simulink model "trainGate"  (R2014b)
settings: Solver=FixedStepDiscrete  StartTime=0.0  StopTime=100000  FixedStep=0.01  MaxStep=0.0001  RelTol=1e-3
settings Model: Creator=sand080  LastModifiedBy=sand080
settings DataIOCC: LimitDataPoints=off

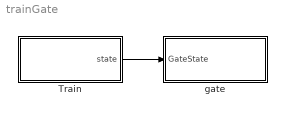
== system trainGate ==
  Train : Subsystem
  gate : Subsystem
  wires:
  Train/1(state) -> gate/1(GateState)

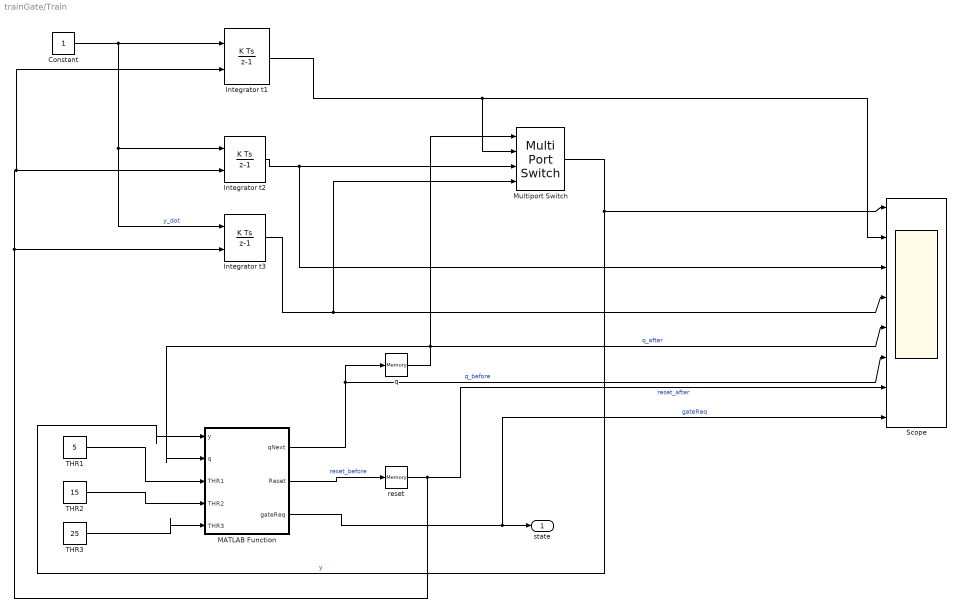
== system trainGate/Train ==
  Constant : Constant
  Integrator t1 : DiscreteIntegrator  ExternalReset=either  InitialConditionSetting=State (most efficient)  SampleTime=-1
  Integrator t2 : DiscreteIntegrator  ExternalReset=either  InitialCondition=5  InitialConditionSetting=State (most efficient)  SampleTime=-1
  Integrator t3 : DiscreteIntegrator  ExternalReset=either  InitialCondition=15  InitialConditionSetting=State (most efficient)  SampleTime=-1
  MATLAB Function : MATLAB Function  Priority=1  TreatAsAtomicUnit=on
  Multiport Switch : MultiPortSwitch
  Scope : Scope  NumInputPorts=8
      settings: TickLabels=on  ShowLegends=on  YMin=0~0~0~10~1~1~0~-1  YMax=40~20~20~30~3~3~1~1
  THR1 : Constant  Value=5
  THR2 : Constant  Value=15
  THR3 : Constant  Value=25
  q : Memory  X0=1  LinearizeMemory=on
  reset : Memory  X0=1  LinearizeMemory=on
  state : Outport
  wires:
  MATLAB Function/1(qNext) -> q/1, Scope/6  "q_before"
  Constant/1 -> Integrator t2/1, Integrator t3/1, Integrator t1/1  "y_dot"
  Integrator t2/1 -> Multiport Switch/3, Scope/3
  Integrator t1/1 -> Scope/2, Multiport Switch/2
  THR1/1 -> MATLAB Function/3(THR1)
  THR2/1 -> MATLAB Function/4(THR2)
  q/1 -> Multiport Switch/1, MATLAB Function/2(q), Scope/5  "q_after"
  THR3/1 -> MATLAB Function/5(THR3)
  Integrator t3/1 -> Multiport Switch/4, Scope/4
  MATLAB Function/2(Reset) -> reset/1  "reset_before"
  Multiport Switch/1 -> Scope/1, MATLAB Function/1(y)  "y"
  reset/1 -> Integrator t1/2, Integrator t2/2, Integrator t3/2, Scope/7  "reset_after"
  MATLAB Function/3(gateReq) -> Scope/8, state/1  "gateReq"

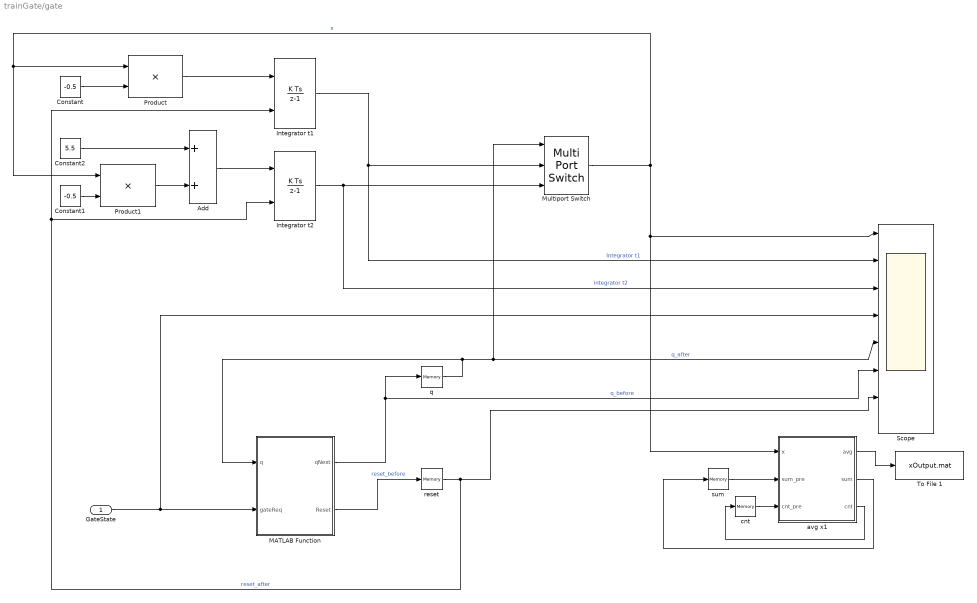
== system trainGate/gate ==
  GateState : Inport
  Add : Sum
  Constant : Constant  Value=-0.5
  Constant1 : Constant  Value=-0.5
  Constant2 : Constant  Value=5.5
  Integrator t1 : DiscreteIntegrator  ExternalReset=either  InitialCondition=10  InitialConditionSetting=State (most efficient)  SampleTime=-1
  Integrator t2 : DiscreteIntegrator  ExternalReset=either  InitialCondition=1  InitialConditionSetting=State (most efficient)  SampleTime=-1
  MATLAB Function : MATLAB Function  Priority=1  TreatAsAtomicUnit=on
  Multiport Switch : MultiPortSwitch  Inputs=2
  Product : Product
  Product1 : Product
  Scope : Scope  NumInputPorts=8
      settings: TickLabels=on  ShowLegends=on  YMin=0~-50~0~-1~1~1~0~-1  YMax=20~50~100~1~2~2~1~1
  To File 1 : ToFile  Filename=xOutput.mat
      settings: Decimation=10000000
  avg x1 : MATLAB Function  Priority=4  TreatAsAtomicUnit=on
  cnt : Memory
  q : Memory  X0=1  LinearizeMemory=on
  reset : Memory  LinearizeMemory=on
  sum : Memory
  wires:
  MATLAB Function/1(qNext) -> q/1, Scope/6  "q_before"
  avg x1/2(sum) -> sum/1
  avg x1/3(cnt) -> cnt/1
  cnt/1 -> avg x1/3(cnt_pre)
  sum/1 -> avg x1/2(sum_pre)
  avg x1/1(avg) -> To File 1/1
  Integrator t2/1 -> Scope/3, Multiport Switch/3  "integrator t2"
  Integrator t1/1 -> Multiport Switch/2, Scope/2  "Integrator t1"
  q/1 -> Multiport Switch/1, Scope/5, MATLAB Function/1(q)  "q_after"
  MATLAB Function/2(Reset) -> reset/1  "reset_before"
  Multiport Switch/1 -> avg x1/1(x), Scope/1, Product/1, Product1/1  "x"
  reset/1 -> Integrator t2/2, Integrator t1/2, Scope/7  "reset_after"
  Constant/1 -> Product/2
  Product/1 -> Integrator t1/1
  Constant1/1 -> Product1/2
  Product1/1 -> Add/2
  Constant2/1 -> Add/1
  Add/1 -> Integrator t2/1
  GateState/1 -> Scope/4, MATLAB Function/2(gateReq)

== matlab function trainGate/gate/MATLAB Function ==
  data: q input; qNext output; Reset output; gateReq input
function [qNext,Reset] = phi(q, gateReq)
%#codegen
if q==1 && gateReq~=1
    qNext=1;
    Reset=0;
elseif q==1 && gateReq==1
    qNext=2;
    Reset=1;
elseif q==2 && gateReq~=-1
    qNext=2;
    Reset=0;
elseif q==2 && gateReq==-1
    qNext=1;
    Reset=1;
else
    qNext=-1; %this should never execute
    Reset=-1; %this should never execute
end

== matlab function trainGate/Train/MATLAB Function ==
  data: y input; q input; qNext output; THR1 input; THR2 input; THR3 input; Reset output; gateReq output
function [qNext,Reset,gateReq] = phi(y,q, THR1, THR2, THR3)
%#codegen
if q==1 && y < THR1
    qNext=1;
    Reset=0;
    gateReq=0;
elseif q==1 && y>=THR1
    qNext=2;
    Reset=1;
    gateReq=1;
elseif q==2 && y<THR2
    qNext=2;
    Reset=0;
    gateReq=0;
elseif q==2 && y>=THR2
    qNext=3;
    Reset=1;
    gateReq=-1;
elseif q==3 && y<THR3
    qNext=3;
    Reset=0;
    gateReq=0;
elseif q==3 && y>=THR3
    qNext=1;
    Reset=1;
    gateReq=0;
else
    qNext=-1; %this should never execute
    Reset=-1; %this should never execute
    gateReq=0;
end

== matlab function trainGate/gate/avg x1 ==
  data: x input; avg output; sum output; cnt output; sum_pre input; cnt_pre input
function [avg, sum,cnt] = fcn(x,  sum_pre, cnt_pre)
%#codegen

cnt=cnt_pre+1;
sum=sum_pre+x;
avg=sum/cnt;
